simulink model "Bode_plot"  (R2023b)
settings: Solver=VariableStepAuto  StartTime=0.0  StopTime=10.0  RelTol=1e-3
values from neighbouring files (symbols this model uses):
  K_d = 0.49    [setup.m]
  K_i = 4.9    [setup.m]
  K_p = 20    [setup.m]
settings Model: Creator=魏浩楠  LastModifiedBy=魏浩楠

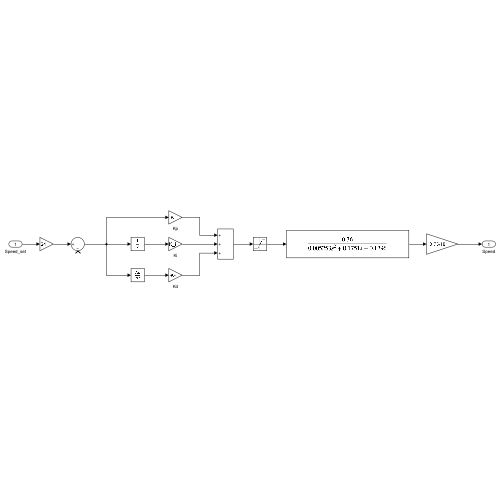
[thumbnail: Simulink's stored preview of the top-level diagram]
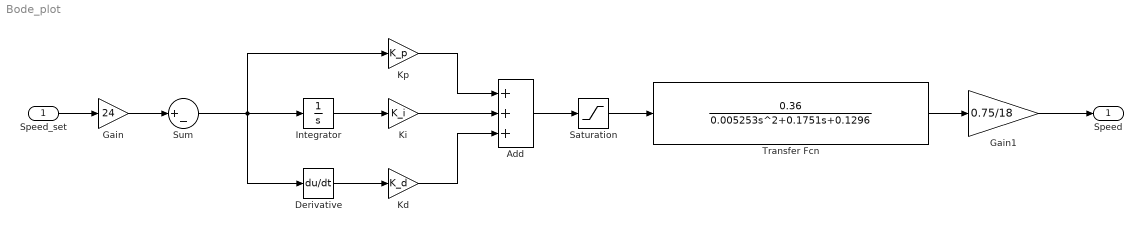
== system Bode_plot ==
  Speed_set : Inport
  Add : Sum  Inputs=+++
  Derivative : Derivative
  Gain : Gain  Gain=24
  Gain1 : Gain  Gain=0.75/18
  Integrator : Integrator
  Kd : Gain  Gain=K_d
  Ki : Gain  Gain=K_i
  Kp : Gain  Gain=K_p
  Saturation : Saturate  UpperLimit=1200  LowerLimit=-1200
  Sum : Sum  Inputs=|+-
  Transfer Fcn : TransferFcn  Numerator=[0.36]  Denominator=[0.005253 0.1751 0.1296]
  Speed : Outport  VectorParamsAs1DForOutWhenUnconnected=off
  wires:
  Saturation/1 -> Transfer Fcn/1
  Kd/1 -> Add/3
  Add/1 -> Saturation/1
  Derivative/1 -> Kd/1
  Transfer Fcn/1 -> Gain1/1
  Kp/1 -> Add/1
  Integrator/1 -> Ki/1
  Sum/1 -> Derivative/1, Kp/1, Integrator/1
  Gain/1 -> Sum/1
  Speed_set/1 -> Gain/1
  Ki/1 -> Add/2
  Gain1/1 -> Speed/1
